simulink model "s_ball_beam_control"  (R2019a)
settings: Solver=ode4  StartTime=0.0  StopTime=25  FixedStep=0.002  RelTol=1e-3  AbsTol=1e-6  EnableMultiTasking=on
values from neighbouring files (symbols this model uses):
  K = 1.53    [setup_ball_beam.m]    (also in setup_ball_beam_OG.m = 10)
  K_bb = 0.418    [setup_ball_beam.m]    (also in setup_ball_beam_OG.m = 1)
  Kc = 5.3    [setup_ball_beam.m]    (also in setup_ball_beam_OG.m = 0.5)
  tau = 0.034    [setup_ball_beam.m]    (also in setup_ball_beam_OG.m = 0.1)
  wf = 2 * pi * 4.0    (= 25.1327412287)    [setup_ball_beam.m]    (also in setup_ball_beam_OG.m)
  z = 1.4    [setup_ball_beam.m]    (also in setup_ball_beam_OG.m = 1)
libraries: simulink_extras x1
settings Model: ExtModeTrigDuration=10000  Creator=MLevis  LastModifiedBy=pmartin
settings SolverCC: AutoScaleAbsTol=off  PositivePriorityOrder=on
settings DataIOCC: SaveFormat=Array  SignalLoggingSaveFormat=ModelDataLogs  ReturnWorkspaceOutputs=off
settings OptimizationCC: BlockReduction=off  BooleanDataType=off  OptimizeBlockIOStorage=off  BufferReuse=off  GlobalBufferReuse=off  ExpressionFolding=off  ExpressionDepthLimit=2147483647  LocalBlockOutputs=off  InitFltsAndDblsToZero=on  LifeSpan=inf  OptimizeDataStoreBuffers=off  BusAssignmentInplaceUpdate=off
settings DebuggingCC: SaveWithParameterizedLinksMsg=none  UnderspecifiedInitializationDetection=Classic  MergeDetectMultiDrivingBlocksExec=none  SignalResolutionControl=TryResolveAllWithWarning  MultiTaskDSMMsg=warning  MultiTaskCondExecSysMsg=none  FcnCallInpInsideContextMsg=warning  StateNameClashWarn=warning  SFUnexpectedBacktrackingDiag=warning  SFNoUnconditionalDefaultTransitionDiag=warning  SFExecutionAtInitializationDiag=none  ArithmeticOperatorsInVariantConditions=warning
settings HardwareCC: ProdBitPerPointer=32  ProdBitPerSizeT=32  ProdBitPerPtrDiffT=32  ProdLargestAtomicFloat=None  ProdIntDivRoundTo=Undefined  ProdEndianess=Unspecified  ProdWordSize=32  ProdHWDeviceType=32-bit Generic  TargetHWDeviceType=32-bit Generic
settings ModelReferenceCC: PropagateSignalLabelsOutOfModel=off
settings RTWCC: SystemTargetFile=quarc_windows.tlc  TemplateMakefile=quarc_default_tmf  Description=Quarc Win32 Target
settings CodeAppCC: StateflowObjectComments=on
settings STFCustomTargetCC: TargetFcnLib=ansi_tfl_tmw.mat  TargetPreCompLibLocation=C:\PROGRA~3\QUARC\lib\2019a\windows\release  ConcurrentExecutionCompliant=on  CPPClassGenCompliant=on  SystemTargetFile=quarc_windows.tlc
settings GRTTargetCC: TargetFcnLib=ansi_tfl_tmw.mat  TargetPreCompLibLocation=C:\PROGRA~3\QUARC\lib\2019a\windows\release  TargetLangStandard=C89/C90 (ANSI)  ParMdlRefBuildCompliant=off  CompOptLevelCompliant=off  CombineOutputUpdateFcns=off  MatFileLogging=off  GRTInterface=on  UseToolchainInfoCompliant=off  ExtMode=on  ExtModeMexFile=quarc_comm
settings ConfigComp: CovMetricSettings=dw  CovHtmlReporting=on  CovSaveCumulativeToWorkspaceVar=on  CovSaveSingleToWorkspaceVar=on

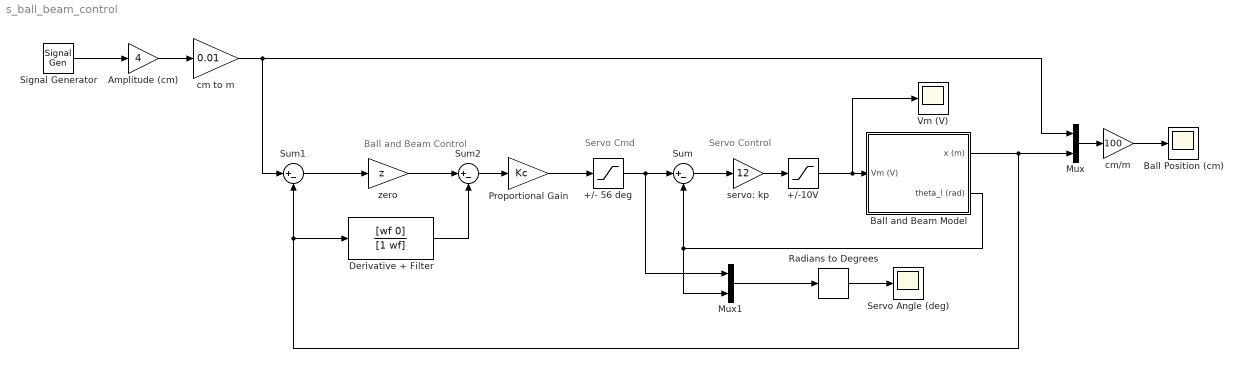
== system s_ball_beam_control ==
  note: Servo Cmd
  note: Ball and Beam Control
  note: Servo Control
  +/- 56 deg : Saturate  UpperLimit=56*pi/180  LowerLimit=-56*pi/180
  +/-10V : Saturate  UpperLimit=10  LowerLimit=-10
  Amplitude (cm) : Gain  Gain=4
  Ball Position (cm) : Scope
  Ball and Beam Model : Subsystem
  Derivative + Filter : TransferFcn  Numerator=[wf 0]  Denominator=[1 wf]
  Mux : Mux  Inputs=2
  Mux1 : Mux  Inputs=2
  Proportional Gain : Gain  Gain=Kc
  Radians to Degrees : simulink_extras/Transformations/Radians to Degrees
  Servo Angle (deg) : Scope
  Signal Generator : SignalGenerator  WaveForm=square  Frequency=0.05
  Sum : Sum  Inputs=|+-
  Sum1 : Sum  Inputs=|+-
  Sum2 : Sum  Inputs=|+-
  Vm (V) : Scope
  cm to m : Gain  Gain=0.01
  cm/m : Gain  Gain=100
  servo: kp : Gain  Gain=12
  zero : Gain  Gain=z
  wires:
  Mux/1 -> cm/m/1
  Amplitude (cm)/1 -> cm to m/1
  Ball and Beam Model/2(theta_l (rad)) -> Mux1/2, Sum/2
  Ball and Beam Model/1(x (m)) -> Mux/2, Derivative + Filter/1, Sum1/2
  Mux1/1 -> Radians to Degrees/1
  cm to m/1 -> Sum1/1, Mux/1
  Radians to Degrees/1 -> Servo Angle (deg)/1
  cm/m/1 -> Ball Position (cm)/1
  Sum/1 -> servo: kp/1
  Sum2/1 -> Proportional Gain/1
  Sum1/1 -> zero/1
  +/- 56 deg/1 -> Sum/1, Mux1/1
  servo: kp/1 -> +/-10V/1
  Proportional Gain/1 -> +/- 56 deg/1
  zero/1 -> Sum2/1
  +/-10V/1 -> Ball and Beam Model/1(Vm (V)), Vm (V)/1
  Signal Generator/1 -> Amplitude (cm)/1
  Derivative + Filter/1 -> Sum2/2

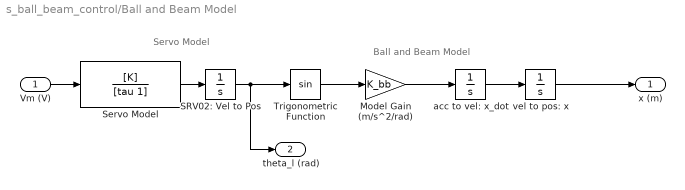
== system s_ball_beam_control/Ball and Beam Model ==
  note: Servo Model
  note: Ball and Beam Model
  Vm (V) : Inport
  Model Gain (m/s^2/rad) : Gain  Gain=K_bb
  SRV02: Vel to Pos : Integrator
  Servo Model : TransferFcn  Numerator=[K]  Denominator=[tau 1]
  Trigonometric Function : Trigonometry
  acc to vel: x_dot : Integrator
  vel to pos: x : Integrator
  x (m) : Outport
  theta_l (rad) : Outport  Port=2
  wires:
  Servo Model/1 -> SRV02: Vel to Pos/1
  Model Gain (m/s^2/rad)/1 -> acc to vel: x_dot/1
  acc to vel: x_dot/1 -> vel to pos: x/1
  Trigonometric Function/1 -> Model Gain (m/s^2/rad)/1
  Vm (V)/1 -> Servo Model/1
  SRV02: Vel to Pos/1 -> Trigonometric Function/1, theta_l (rad)/1
  vel to pos: x/1 -> x (m)/1
